simulink model "VSG_10k"  (R2022b)
settings: Solver=FixedStepAuto  StartTime=0.0  StopTime=4  FixedStep=1e-6  RelTol=1e-3
model workspace (MAT data in the model file):
  C = 0.0002
  D = 100
  GP = 1
  GQ = 3
  J = 5
  KQ = 0.06
  Kf = 120
  Kv = 577
  L = 0.002
  Pref = 10000
  Qref = 0
  Ts = 1e-06
  Ug = 563.38264084
  Vdc = 800
  fsw = 20000
  t0 = 0.5
  tco = 1.3
  tf = 1.2
  wn = 314.159265359
undefined symbols (not defined in the file): DiscIntNeverNeededParam
libraries: spsabctodq0Lib x4, spsPowerPositiveSequenceLib x4, slpidlib x4, spsFirstOrderFilterLib x3, spsMultimeterLib x3, spsThreePhaseSeriesRLCBranchLib x3, spsThreePhaseVIMeasurementLib x3, spsGroundLib x2, spsPLL3phLib x2, spsDCVoltageSourceLib x1, spsPWMGenerator2LevelLib x1, spsdq0toabcLib x1
settings Model: SimulationMode=accelerator  Creator=刘明炜  LastModifiedBy=user
settings DataIOCC: ReturnWorkspaceOutputs=off

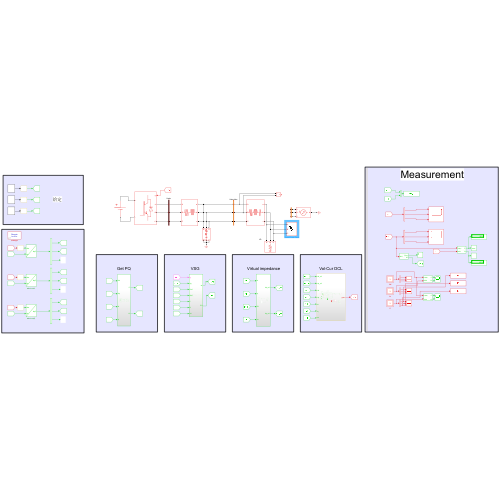
[thumbnail: Simulink's stored preview of the top-level diagram]
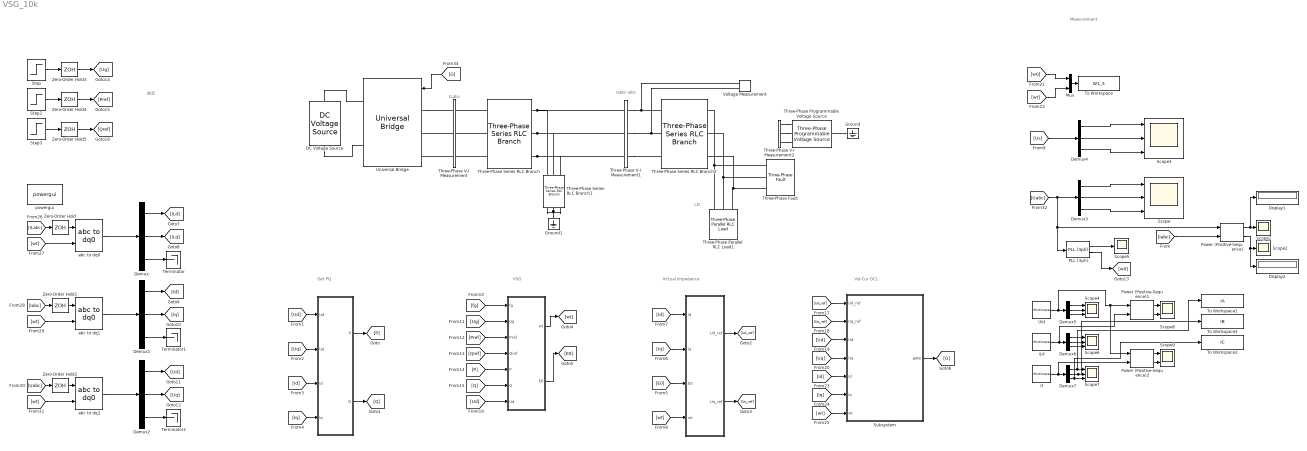
== system VSG_10k ==
  note: Measurement
  note: 给定
  note: ILabc
  note: VSG
  note: LD
  note: Get PQ
  note: Virtual impedance
  note: Vol-Cur DCL
  note: Uabc-Iabc
  " " : Subsystem
  "  " : Subsystem
  "   " : Subsystem
  DC Voltage Source : spsDCVoltageSourceLib/DC Voltage Source  Amplitude=1000  Measurements=None
  Demux{,1..7} (8 alike) : Demux  Outputs=3
  Display1 : Display
  Display2 : Display
  Ground : spsGroundLib/Ground  LConnTagsString=a
  Ground1 : spsGroundLib/Ground  LConnTagsString=a
  If : spsMultimeterLib/Multimeter  L=12  sel=[10 11 12]  yselected={}  Gain=[1 1 1]  OutputType=Complex  PlotAtSimulationStop=off  PhasorSimulation=off
  Mux : Mux  Inputs=2
  PLL (3ph) : spsPLL3phLib/PLL (3ph)  Fmin=45  Par_Init=[0, 50]  ParK=[180, 3200, 1]  TcD=1e-4  MaxRateChangeFreq=12  FilterCutOffFreq=25  Ts=1/fsw  AGC=on
  Power (Positive-Sequence) : spsPowerPositiveSequenceLib/Power (Positive-Sequence)  Freq=50  Vinit=[0, 0]  Iinit=[0, 0]  Ts=1/fsw
      settings: LibrarySourceBlock=|
      | sps_lib/Sensors and Measurements/Power
      | (Positive-Sequence)
  Power (Positive-Sequence)1 : spsPowerPositiveSequenceLib/Power (Positive-Sequence)  Freq=50  Vinit=[0, 0]  Iinit=[0, 0]  Ts=1/fsw
      settings: LibrarySourceBlock=|
      | sps_lib/Sensors and Measurements/Power
      | (Positive-Sequence)
  Power (Positive-Sequence)2 : spsPowerPositiveSequenceLib/Power (Positive-Sequence)  Freq=50  Vinit=[0, 0]  Iinit=[0, 0]  Ts=1/fsw
      settings: LibrarySourceBlock=|
      | sps_lib/Sensors and Measurements/Power
      | (Positive-Sequence)
  Scope{,3..4,6..7} (5 alike) : Scope  NumInputPorts=3
  Scope1 : Scope
  Scope2 : Scope
  Scope5 : Scope
  Scope8 : Scope  NumInputPorts=2
  Scope9 : Scope  NumInputPorts=2
  Step : Step  Time=0.5  Before=1  After=Ug  SampleTime=0
  Step1 : Step  Time=t0  After=Pref  SampleTime=0
  Step3 : Step  Time=t0  After=Qref  SampleTime=0
  Subsystem : Subsystem
  Terminator : Terminator
  Terminator1 : Terminator
  Terminator2 : Terminator
  Three-Phase Parallel RLC Load1 : spsThreePhaseParallelRLCLoadLib/Three-Phase Parallel RLC Load  LConnTagsString=A|B|C  Configuration=Y (grounded)  NominalVoltage=690  Vabc=[1e3 1e3 1e3]  Vabcp=[1e3 1e3 1e3]  NominalFrequency=50  UnbalancedPower=off  ActivePower=10e3  InductivePower=0  CapacitivePower=0  Pabc=[10e3 9e3 11e3]  QLabc=[100 90 110]  QCabc=[100 90 110]  Pabcp=[10e3 9e3 11e3]  QLabcp=[100 90 110]  QCabcp=[100 90 110]  Measurements=Branch voltages and currents  LoadType=constant Z
  Three-Phase Programmable Voltage Source : spsThreePhaseProgrammableVoltageSourceLib/Three-Phase Programmable Voltage Source  PositiveSequence="[690  0 50]"  VariationEntity=None  VariationType=Table of time-amplitude pairs  VariationTypeAlt=Step  VariationStep=0.5  VariationRate=10  VariationMagnitude=0.3  VariationFrequency=2  VariationTiming=[1 2]  VariationPhaseA=off  Amplitudes=[1 0.8 1.2 1.0]  TimeValues=[0 0.1 0.15 0.2]  HarmonicGeneration=off  HarmonicA=[3 0.2 -25 0]  HarmonicB=[2 0.15 35 2]  Timing="[0.05  3]"  BusType=PQ  Pref=-20000  Qref=0  Qmin=-inf  Qmax=inf
  Three-Phase Series RLC Branch : spsThreePhaseSeriesRLCBranchLib/Three-Phase Series RLC Branch  LConnTagsString=A|B|C  RConnTagsString=A|B|C  BranchType=RL  Resistance=0  Inductance=0.002  Capacitance=0  Measurements=None
  Three-Phase Series RLC Branch1 : spsThreePhaseSeriesRLCBranchLib/Three-Phase Series RLC Branch  LConnTagsString=A|B|C  RConnTagsString=A|B|C  BranchType=RLC  Resistance=1  Inductance=0  Capacitance=0.0002  Measurements=None
  Three-Phase Series RLC Branch2 : spsThreePhaseSeriesRLCBranchLib/Three-Phase Series RLC Branch  LConnTagsString=A|B|C  RConnTagsString=A|B|C  BranchType=RLC  Resistance=0  Inductance=7e-3  Capacitance=0  Measurements=None
  Three-Phase V-I Measurement : spsThreePhaseVIMeasurementLib/Three-Phase V-I Measurement  VoltageMeasurement=phase-to-phase  SetLabelV=on  LabelV=vnon  Vpu=off  VpuLL=off  CurrentMeasurement=yes  SetLabelI=on  LabelI=ILabc  Ipu=off  Pbase=100e6  Vbase=500e3  OutputType=Complex  PhasorSimulation=off  PSBequivalent=0
  Three-Phase V-I Measurement1 : spsThreePhaseVIMeasurementLib/Three-Phase V-I Measurement  VoltageMeasurement=phase-to-ground  SetLabelV=on  LabelV=Uabc  Vpu=off  VpuLL=off  CurrentMeasurement=yes  SetLabelI=on  LabelI=Iabc  Ipu=off  Pbase=100e6  Vbase=500e3  OutputType=Complex  PhasorSimulation=off  PSBequivalent=0
  Three-Phase V-I Measurement2 : spsThreePhaseVIMeasurementLib/Three-Phase V-I Measurement  VoltageMeasurement=phase-to-ground  SetLabelV=on  LabelV=Us  Vpu=off  VpuLL=off  CurrentMeasurement=yes  SetLabelI=on  LabelI=Is  Ipu=off  Pbase=100e6  Vbase=500e3  OutputType=Complex  PhasorSimulation=off  PSBequivalent=0
  Three-Phase Fault : spsThreePhaseFaultLib/Three-Phase Fault  InitialStates=0  FaultA=on  FaultB=off  FaultC=off  GroundFault=on  SwitchTimes="[tf  tco]"  External=off  SwitchStatus=NaN  FaultResistance=0.001  GroundResistance=0.01  SnubberResistance=1e6  SnubberCapacitance=inf  Measurements=Fault voltages and currents
  To Workspace : ToWorkspace  VariableName=W1_5  SaveFormat=Timeseries  SampleTime=-1
  To Workspace1 : ToWorkspace  VariableName=IA  SaveFormat=Timeseries  SampleTime=-1
  To Workspace2 : ToWorkspace  VariableName=IC  SaveFormat=Timeseries  SampleTime=-1
  To Workspace3 : ToWorkspace  VariableName=IB  SaveFormat=Timeseries  SampleTime=-1
  Uld : spsMultimeterLib/Multimeter  L=12  sel=[1 2 3]  yselected={}  Gain=[1 1 1]  OutputType=Complex  PlotAtSimulationStop=off  PhasorSimulation=off
  Universal Bridge : spsUniversalBridgeLib/Universal Bridge  Arms=3  SnubberResistance=1e5  SnubberCapacitance=inf  Device=IGBT / Diodes  Ron=0.001  Lon=0  ForwardVoltages="[  0  0  ]"  ForwardVoltage=0  GTOparameters=[ 10e-6 , 20e-6 ]  IGBTparameters=[ 1e-6 , 2e-6 ]  Measurements=None  Measurements_2=None  converterType=Rectifier
  Voltage Measurement : spsVoltageMeasurementLib/Voltage Measurement  PhasorSimulation=off  OutputType=Complex  PSBequivalent=0
  Zero-Order Hold{,1..5} (6 alike) : ZeroOrderHold  SampleTime=1/fsw
  abc to dq0 : spsabctodq0Lib/abc to dq0  Alignment=90 degrees behind phase A axis
  abc to dq1 : spsabctodq0Lib/abc to dq0  Alignment=90 degrees behind phase A axis
  abc to dq2 : spsabctodq0Lib/abc to dq0  Alignment=90 degrees behind phase A axis
  iLd : spsMultimeterLib/Multimeter  L=12  sel=[7 8 9]  yselected={}  Gain=[1 1 1]  OutputType=Complex  PlotAtSimulationStop=off  PhasorSimulation=off
  powergui : sps_lib/powergui  Priority=1  SimulationMode=Discrete  SampleTime=1e-6  frequency=60  Iterations=50  frequencyindice=0  Pbase=100e6  ErrMax=1e-4  UnitsV=kV  UnitsW=MW  buscounter=0  FunctionMessages=off  echomessages=off  EnableUseOfTLC=off  CurrentSourceSwitches=off  DisableSnubberDevices=off  DisableRonSwitches=off  DisableVfSwitches=off  DisplayEquations=off  AutomaticDiscreteSolvers=off  SolverType=Tustin/Backward Euler (TBE)  Interpol=off  ExternalGateDelay=off  methode=off  Ts=100  x0status=blocks  SPID=on  SwTol=0  HookPort=off  NonlinearTolerance=1e-4  nMaxIteration=100  ContinueOnMaxIteration=off  RestoreLinks=warning  ResistiveCurrentMeasurement=off  Frange=[0:2:500]  Ylog=off  Xlog=on  ShowGrid=off  save=off  variable=ZData  structure=0  ZoomFFT=off  StartTime=0.0  cycles=1  DisplayStyle=1  fundamental=60  FreqAxis=off  MaxFrequency=1000  frequencyindicesteady=1  RmsSteady=1  display=off
  wires:
  [Id] -> " "/3(Id)
  [Iq] -> " "/4(Iq)
  [Uq] -> " "/2(Uq)
  " "/1(P) -> [P]
  [Ud] -> " "/1(Ud)
  " "/2(Q) -> [Q]
  [E0] -> "   "/3(E0)
  [Iq] -> "   "/2(Iq)
  [Id] -> "   "/1(Id)
  [wt] -> "   "/4(wt)
  "   "/1(Ud_ref) -> [Ud_ref]
  "   "/2(Uq_ref) -> [Uq_ref]
  [Qref] -> "  "/4(Qref)
  [Ud] -> "  "/7(Ud)
  [fg] -> "  "/1(fg)
  "  "/2(E0) -> [E0]
  [Q] -> "  "/6(Q)
  [P] -> "  "/5(P)
  [Ug] -> "  "/2(Ug)
  [Pref] -> "  "/3(Pref)
  "  "/1(wt) -> [wt]
  [Ud] -> Subsystem/3(Ud)
  Subsystem/1(gate) -> [G]
  [wt] -> Subsystem/7(wt)
  [Ud_ref] -> Subsystem/1(Ud_ref)
  [Uq_ref] -> Subsystem/2(Uq_ref)
  [Iq] -> Subsystem/6(Iq)
  [Uq] -> Subsystem/4(Uq)
  [Id] -> Subsystem/5(Id)
  abc to dq0/1 -> Demux/1
  Demux/1 -> [ILd]
  Demux/2 -> [ILq]
  Demux/3 -> Terminator/1
  Demux1/2 -> [Iq]
  Demux1/1 -> [Id]
  abc to dq1/1 -> Demux1/1
  Demux1/3 -> Terminator1/1
  Demux2/2 -> [Uq]
  Demux2/1 -> [Ud]
  abc to dq2/1 -> Demux2/1
  Demux2/3 -> Terminator2/1
  Zero-Order Hold/1 -> abc to dq0/1
  [ILabc] -> Zero-Order Hold/1
  [Iabc] -> Zero-Order Hold1/1
  Zero-Order Hold1/1 -> abc to dq1/1
  [Uabc] -> Zero-Order Hold2/1
  Zero-Order Hold2/1 -> abc to dq2/1
  [wt] -> abc to dq0/2
  [wt] -> abc to dq1/2
  [wt] -> abc to dq2/2
  Step/1 -> Zero-Order Hold3/1
  Zero-Order Hold3/1 -> [Ug]
  Zero-Order Hold4/1 -> [Pref]
  Step1/1 -> Zero-Order Hold4/1
  [Uabc] -> PLL (3ph)/1, Power (Positive-Sequence)/1, Demux3/1
  Demux3/1 -> Scope/1
  Demux3/2 -> Scope/2
  Demux3/3 -> Scope/3
  [G] -> Universal Bridge/1
  [Iabc] -> Power (Positive-Sequence)/2
  Power (Positive-Sequence)/1 -> Display1/1, Scope1/1
  Power (Positive-Sequence)/2 -> Display2/1, Scope2/1
  Step3/1 -> Zero-Order Hold5/1
  Zero-Order Hold5/1 -> [Qref]
  Demux4/2 -> Scope3/2
  Demux4/3 -> Scope3/3
  [Us] -> Demux4/1
  Demux4/1 -> Scope3/1
  PLL (3ph)/1 -> Scope5/1
  PLL (3ph)/2 -> [w0]
  [w0] -> Mux/1
  [wt] -> Mux/2
  Mux/1 -> To Workspace/1
  Uld/1 -> Power (Positive-Sequence)2/1, Power (Positive-Sequence)1/1, Demux5/1
  iLd/1 -> Power (Positive-Sequence)1/2, Demux6/1
  If/1 -> Power (Positive-Sequence)2/2, Demux7/1
  Demux5/1 -> Scope4/1
  Demux5/2 -> Scope4/2
  Demux5/3 -> Scope4/3
  Demux6/1 -> Scope6/1
  Demux6/2 -> Scope6/2
  Demux6/3 -> Scope6/3
  Demux7/1 -> To Workspace1/1, Scope7/1
  Demux7/2 -> To Workspace3/1, Scope7/2
  Demux7/3 -> To Workspace2/1, Scope7/3
  Power (Positive-Sequence)1/1 -> Scope8/1
  Power (Positive-Sequence)1/2 -> Scope8/2
  Power (Positive-Sequence)2/1 -> Scope9/1
  Power (Positive-Sequence)2/2 -> Scope9/2
  connections:
  Three-Phase Series RLC Branch/RConn1 -- Three-Phase V-I Measurement1/LConn1 -- Three-Phase Series RLC Branch1/LConn1
  Ground1/LConn1 -- Three-Phase Series RLC Branch1/RConn2 -- Three-Phase Series RLC Branch1/RConn3 -- Three-Phase Series RLC Branch1/RConn1
  Three-Phase Series RLC Branch/RConn3 -- Three-Phase V-I Measurement1/LConn3 -- Three-Phase Series RLC Branch1/LConn3
  Three-Phase Series RLC Branch/RConn2 -- Three-Phase Series RLC Branch1/LConn2 -- Three-Phase V-I Measurement1/LConn2
  Three-Phase Series RLC Branch/LConn1 -- Three-Phase V-I Measurement/RConn1
  Three-Phase V-I Measurement1/RConn3 -- Three-Phase Series RLC Branch2/LConn3
  Three-Phase V-I Measurement/LConn2 -- Universal Bridge/LConn2
  DC Voltage Source/LConn1 -- Universal Bridge/RConn2
  Universal Bridge/LConn1 -- Three-Phase V-I Measurement/LConn1
  Three-Phase V-I Measurement1/RConn2 -- Voltage Measurement/LConn2 -- Three-Phase Series RLC Branch2/LConn2
  DC Voltage Source/RConn1 -- Universal Bridge/RConn1
  Three-Phase V-I Measurement1/RConn1 -- Voltage Measurement/LConn1 -- Three-Phase Series RLC Branch2/LConn1
  Three-Phase Series RLC Branch/LConn2 -- Three-Phase V-I Measurement/RConn2
  Three-Phase Series RLC Branch/LConn3 -- Three-Phase V-I Measurement/RConn3
  Three-Phase V-I Measurement/LConn3 -- Universal Bridge/LConn3
  Ground/LConn1 -- Three-Phase Programmable Voltage Source/LConn1
  Three-Phase V-I Measurement2/RConn1 -- Three-Phase Programmable Voltage Source/RConn1
  Three-Phase V-I Measurement2/RConn2 -- Three-Phase Programmable Voltage Source/RConn2
  Three-Phase V-I Measurement2/RConn3 -- Three-Phase Programmable Voltage Source/RConn3
  Three-Phase Parallel RLC Load1/LConn1 -- Three-Phase Fault/LConn1 -- Three-Phase Series RLC Branch2/RConn1
  Three-Phase Parallel RLC Load1/LConn3 -- Three-Phase Series RLC Branch2/RConn3 -- Three-Phase Fault/LConn3
  Three-Phase Fault/LConn2 -- Three-Phase Series RLC Branch2/RConn2 -- Three-Phase Parallel RLC Load1/LConn2

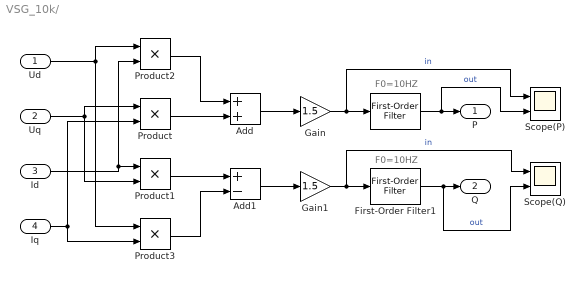
== system VSG_10k/  ==
  note: F0=10HZ
  note: F0=10HZ
  Ud : Inport
  Uq : Inport  Port=2
  Id : Inport  Port=3
  Iq : Inport  Port=4
  " " : spsFirstOrderFilterLib/First-Order Filter  FilterType=Lowpass  Tc=10e-3  Ts=1/fsw  Initialize=on  Vac_Init=[0, 0, 10]  Vdc_Init=0  PlotResponse=off  FreqRange="[0,  200,  1]"
  Add : Sum
  Add1 : Sum  Inputs=+-
  First-Order Filter1 : spsFirstOrderFilterLib/First-Order Filter  FilterType=Lowpass  Tc=10e-3  Ts=1/fsw  Initialize=on  Vac_Init=[0, 0, 10]  Vdc_Init=0  PlotResponse=off  FreqRange="[0,  200,  1]"
  Gain : Gain  Gain=1.5
  Gain1 : Gain  Gain=1.5
  Product{,1..3} (4 alike) : Product
  Scope(P) : Scope  NumInputPorts=2
  Scope(Q) : Scope  NumInputPorts=2
  P : Outport
  Q : Outport  Port=2
  wires:
  Gain1/1 -> First-Order Filter1/1, Scope(Q)/1  "in"
  Product2/1 -> Add/1
  " "/1 -> Scope(P)/2, P/1  "out"
  Add1/1 -> Gain1/1
  Gain/1 -> " "/1, Scope(P)/1  "in"
  First-Order Filter1/1 -> Scope(Q)/2, Q/1  "out"
  Product/1 -> Add/2
  Product3/1 -> Add1/2
  Product1/1 -> Add1/1
  Ud/1 -> Product3/1, Product2/1
  Add/1 -> Gain/1
  Id/1 -> Product1/1, Product2/2
  Iq/1 -> Product3/2, Product/2
  Uq/1 -> Product1/2, Product/1

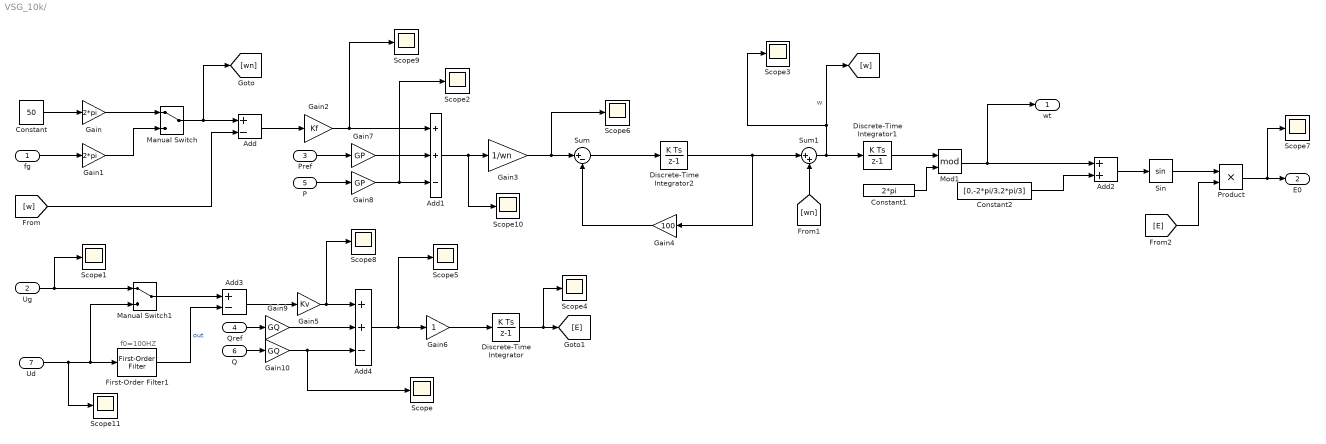
== system VSG_10k/   ==
  note: f0=100HZ
  note: w
  fg : Inport
  Ug : Inport  Port=2
  Pref : Inport  Port=3
  Qref : Inport  Port=4
  P : Inport  Port=5
  Q : Inport  Port=6
  Ud : Inport  Port=7
  Add : Sum  Inputs=+-
  Add1 : Sum  Inputs=++-
  Add2 : Sum
  Add3 : Sum  Inputs=+-
  Add4 : Sum  Inputs=++-
  Constant : Constant  Value=50
  Constant1 : Constant  Value=2*pi
  Constant2 : Constant  Value=[0,-2*pi/3,2*pi/3]
  Discrete-Time Integrator : DiscreteIntegrator  gainval=KQ  SampleTime=1/fsw  ICPrevOutput=DiscIntNeverNeededParam  ICPrevScaledInput=DiscIntNeverNeededParam
  Discrete-Time Integrator1 : DiscreteIntegrator  SampleTime=1/fsw  ICPrevOutput=DiscIntNeverNeededParam  ICPrevScaledInput=DiscIntNeverNeededParam
  Discrete-Time Integrator2 : DiscreteIntegrator  gainval=1/J  SampleTime=1/fsw  ICPrevOutput=DiscIntNeverNeededParam  ICPrevScaledInput=DiscIntNeverNeededParam
  First-Order Filter1 : spsFirstOrderFilterLib/First-Order Filter  FilterType=Lowpass  Tc=10e-3  Ts=1/fsw  Initialize=on  Vac_Init=[0, 0, 10]  Vdc_Init=0  PlotResponse=off  FreqRange="[0,  200,  1]"
  Gain : Gain  Gain=2*pi
  Gain1 : Gain  Gain=2*pi
  Gain10 : Gain  Gain=GQ
  Gain2 : Gain  Gain=Kf
  Gain3 : Gain  Gain=1/wn
  Gain4 : Gain  Gain=100
  Gain5 : Gain  Gain=Kv
  Gain6 : Gain
  Gain7 : Gain  Gain=GP
  Gain8 : Gain  Gain=GP
  Gain9 : Gain  Gain=GQ
  Manual Switch : ManualSwitch
  Manual Switch1 : ManualSwitch
  Mod1 : Math  Operator=mod
  Product : Product
  Scope{,1..11} (12 alike) : Scope
  Sin : Trigonometry
  Sum : Sum  Inputs=|+-
  Sum1 : Sum  Inputs=|++
  wt : Outport
  E0 : Outport  Port=2
  wires:
  Ug/1 -> Scope1/1, Manual Switch1/1
  Gain3/1 -> Scope6/1, Sum/1
  Gain2/1 -> Scope9/1, Add1/1
  Product/1 -> Scope7/1, E0/1
  Add/1 -> Gain2/1
  Manual Switch1/1 -> Add3/1
  [E] -> Product/2
  Add4/1 -> Scope5/1, Gain6/1
  Mod1/1 -> wt/1, Add2/1
  Sum1/1 -> Discrete-Time Integrator1/1, Scope3/1, [w]
  fg/1 -> Gain1/1
  Constant2/1 -> Add2/2
  First-Order Filter1/1 -> Add3/2  "out"
  Constant/1 -> Gain/1
  Sin/1 -> Product/1
  Add2/1 -> Sin/1
  Gain4/1 -> Sum/2
  P/1 -> Gain8/1
  Gain/1 -> Manual Switch/1
  Gain1/1 -> Manual Switch/2
  Discrete-Time Integrator2/1 -> Gain4/1, Sum1/1
  Constant1/1 -> Mod1/2
  Gain5/1 -> Scope8/1, Add4/1
  Q/1 -> Gain10/1
  Manual Switch/1 -> [wn], Add/1
  Pref/1 -> Gain7/1
  Add1/1 -> Scope10/1, Gain3/1
  Add3/1 -> Gain5/1
  Gain6/1 -> Discrete-Time Integrator/1
  Qref/1 -> Gain9/1
  [wn] -> Sum1/2
  Sum/1 -> Discrete-Time Integrator2/1
  Discrete-Time Integrator/1 -> Scope4/1, [E]
  Discrete-Time Integrator1/1 -> Mod1/1
  [w] -> Add/2
  Gain7/1 -> Add1/2
  Gain8/1 -> Scope2/1, Add1/3
  Gain9/1 -> Add4/2
  Gain10/1 -> Scope/1, Add4/3
  Ud/1 -> Scope11/1, First-Order Filter1/1, Manual Switch1/2

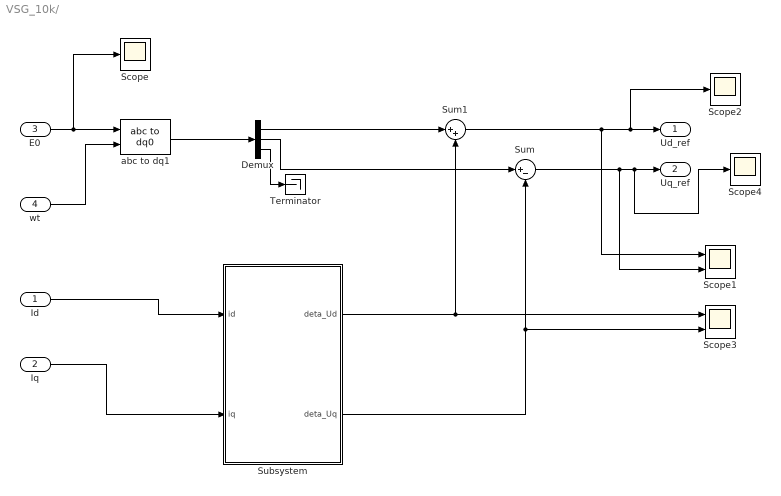
== system VSG_10k/    ==
  Id : Inport
  Iq : Inport  Port=2
  E0 : Inport  Description=Cont  Port=3
  wt : Inport  Port=4
  Demux : Demux  Outputs=3
  Scope : Scope
  Scope1 : Scope  NumInputPorts=2
  Scope2 : Scope
  Scope3 : Scope  NumInputPorts=2
  Scope4 : Scope
  Subsystem : Subsystem
  Sum : Sum  Inputs=|+-
  Sum1 : Sum  Inputs=|++
  Terminator : Terminator
  abc to dq1 : spsabctodq0Lib/abc to dq0  Alignment=90 degrees behind phase A axis
  Ud_ref : Outport
  Uq_ref : Outport  Port=2
  wires:
  Demux/1 -> Sum1/1
  E0/1 -> Scope/1, abc to dq1/1
  Id/1 -> Subsystem/1(id)
  abc to dq1/1 -> Demux/1
  Subsystem/2(deta_Uq) -> Scope3/2, Sum/2
  Sum1/1 -> Scope2/1, Ud_ref/1, Scope1/1
  wt/1 -> abc to dq1/2
  Demux/2 -> Sum/1
  Subsystem/1(deta_Ud) -> Sum1/2, Scope3/1
  Iq/1 -> Subsystem/2(iq)
  Sum/1 -> Scope4/1, Uq_ref/1, Scope1/2
  Demux/3 -> Terminator/1

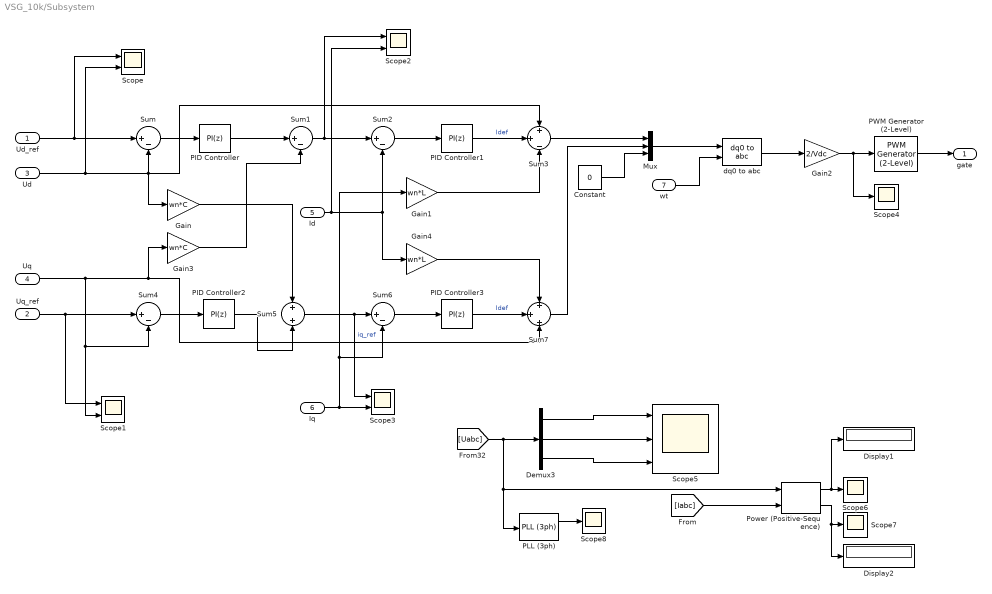
== system VSG_10k/Subsystem ==
  Ud_ref : Inport
  Uq_ref : Inport  Port=2
  Ud : Inport  Port=3
  Uq : Inport  Port=4
  Id : Inport  Port=5
  Iq : Inport  Port=6
  wt : Inport  Port=7
  Constant : Constant  Value=0
  Demux3 : Demux  Outputs=3
  Display1 : Display
  Display2 : Display
  Gain : Gain  Gain=wn*C
  Gain1 : Gain  Gain=wn*L
  Gain2 : Gain  Gain=2/Vdc
  Gain3 : Gain  Gain=wn*C
  Gain4 : Gain  Gain=wn*L
  Mux : Mux  Inputs=3
  PID Controller : slpidlib/PID Controller  Controller=PI  Form=Parallel  TimeDomain=Discrete-time  UseExternalTs=off  SampleTime=-1  IntegratorMethod=Forward Euler  FilterMethod=Forward Euler  ControllerParametersSource=internal  P=10  I=50  UseKiTs=off  D=0  N=100  UseFilter=on  TunerSelectOption=Transfer Function Based (PID Tuner App)  InitialConditionSource=internal  InitialConditionForIntegrator=0  InitialConditionForFilter=0  DifferentiatorICPrevScaledInput=0  ExternalReset=none  TrackingMode=off  Kt=1  LimitOutput=off  SatLimitsSource=internal  UpperSaturationLimit=inf  LowerSaturationLimit=-inf  LinearizeAsGain=on  AntiWindupMode=none  Kb=1  LimitIntegrator=off  UpperIntegratorSaturationLimit=inf  LowerIntegratorSaturationLimit=-inf  POutMin=[]  POutMax=[]  IOutMin=[]  IOutMax=[]  DOutMin=[]  DOutMax=[]  NOutMin=[]  NOutMax=[]  SumOutMin=[]  SumOutMax=[]  SaturationOutMin=[]  SaturationOutMax=[]  PParamMin=[]  PParamMax=[]  IParamMin=[]  IParamMax=[]  DParamMin=[]  DParamMax=[]  NParamMin=[]  NParamMax=[]  KbParamMin=[]  KbParamMax=[]  KtParamMin=[]  KtParamMax=[]  KbOutMin=[]  KbOutMax=[]  KtOutMin=[]  KtOutMax=[]  IntegratorOutMin=[]  IntegratorOutMax=[]  FilterOutMin=[]  FilterOutMax=[]  SumI1OutMin=[]  SumI1OutMax=[]  SumI2OutMin=[]  SumI2OutMax=[]  SumI3OutMin=[]  SumI3OutMax=[]  SumI4OutMin=[]  SumI4OutMax=[]  SumDOutMin=[]  SumDOutMax=[]  DifferentiatorOutMin=[]  DifferentiatorOutMax=[]  FilterDiffOutCoefMin=[]  FilterDiffOutCoefMax=[]  ReciprocalOutMin=[]  ReciprocalOutMax=[]  SumDenOutMin=[]  SumDenOutMax=[]  SumNumOutMin=[]  SumNumOutMax=[]  DivideOutMin=[]  DivideOutMax=[]  UdiffTsProdOutMin=[]  UdiffTsProdOutMax=[]  NTsProdOutMin=[]  NTsProdOutMax=[]  UintegralTsProdOutMin=[]  UintegralTsProdOutMax=[]  UngainTsProdOutMin=[]  UngainTsProdOutMax=[]  ClampingZeroOutDataTypeStr=Inherit: Inherit via back propagation  ClampingZeroOutMin=[]  ClampingZeroOutMax=[]  FilterDenConstantOutDataTypeStr=Inherit: Inherit via back propagation  FilterDenConstantOutMin=[]  FilterDenConstantOutMax=[]  PCopyOutDataTypeStr=Inherit: Inherit via back propagation  PCopyOutMin=[]  PCopyOutMax=[]  NCopyOutDataTypeStr=Inherit: Inherit via back propagation  NCopyOutMin=[]  NCopyOutMax=[]  IntegratorContinuousStateAttributes=''  IntegratorStateMustResolveToSignalObject=off  IntegratorRTWStateStorageClass=Auto  FilterContinuousStateAttributes=''  FilterStateMustResolveToSignalObject=off  FilterRTWStateStorageClass=Auto  ParallelPVariant=InternalParameters  IdealPVariant=Disabled  IVariant=InternalParameters  DVariant=Disabled  IntegratorVariant=Discrete  SatVariant=Disabled  AWVariant=Passthrough  PCopyVariant=Disabled  TRVariant=Disabled  FdbkBlocksVariant=Forward  IdealPFdbkVariant=Disabled  SatFdbkVariant=Disabled  DerivativeFilterVariant=Disabled  NVariant=Disabled  NCopyVariant=Disabled_SignalSpec  FilterICVariant=Disabled  IntegratorICVariant=InternalICs  ExternalResetVariant=Disabled  TRSumVariant=Passthrough  SumFdbkVariant=Disabled  SumVariant=Sum_PI  TsampFilterVariant=InternalTs  TsampNgainVariant=Passthrough  TsampIntegralVariant=Passthrough  ExternalSaturationOutDataTypeStr=Inherit: Same as second input
  PID Controller1 : slpidlib/PID Controller  Controller=PI  Form=Parallel  TimeDomain=Discrete-time  UseExternalTs=off  SampleTime=-1  IntegratorMethod=Forward Euler  FilterMethod=Forward Euler  ControllerParametersSource=internal  P=20  I=50  UseKiTs=off  D=0  N=100  UseFilter=on  TunerSelectOption=Transfer Function Based (PID Tuner App)  InitialConditionSource=internal  InitialConditionForIntegrator=0  InitialConditionForFilter=0  DifferentiatorICPrevScaledInput=0  ExternalReset=none  TrackingMode=off  Kt=1  LimitOutput=off  SatLimitsSource=internal  UpperSaturationLimit=inf  LowerSaturationLimit=-inf  LinearizeAsGain=on  AntiWindupMode=none  Kb=1  LimitIntegrator=off  UpperIntegratorSaturationLimit=inf  LowerIntegratorSaturationLimit=-inf  POutMin=[]  POutMax=[]  IOutMin=[]  IOutMax=[]  DOutMin=[]  DOutMax=[]  NOutMin=[]  NOutMax=[]  SumOutMin=[]  SumOutMax=[]  SaturationOutMin=[]  SaturationOutMax=[]  PParamMin=[]  PParamMax=[]  IParamMin=[]  IParamMax=[]  DParamMin=[]  DParamMax=[]  NParamMin=[]  NParamMax=[]  KbParamMin=[]  KbParamMax=[]  KtParamMin=[]  KtParamMax=[]  KbOutMin=[]  KbOutMax=[]  KtOutMin=[]  KtOutMax=[]  IntegratorOutMin=[]  IntegratorOutMax=[]  FilterOutMin=[]  FilterOutMax=[]  SumI1OutMin=[]  SumI1OutMax=[]  SumI2OutMin=[]  SumI2OutMax=[]  SumI3OutMin=[]  SumI3OutMax=[]  SumI4OutMin=[]  SumI4OutMax=[]  SumDOutMin=[]  SumDOutMax=[]  DifferentiatorOutMin=[]  DifferentiatorOutMax=[]  FilterDiffOutCoefMin=[]  FilterDiffOutCoefMax=[]  ReciprocalOutMin=[]  ReciprocalOutMax=[]  SumDenOutMin=[]  SumDenOutMax=[]  SumNumOutMin=[]  SumNumOutMax=[]  DivideOutMin=[]  DivideOutMax=[]  UdiffTsProdOutMin=[]  UdiffTsProdOutMax=[]  NTsProdOutMin=[]  NTsProdOutMax=[]  UintegralTsProdOutMin=[]  UintegralTsProdOutMax=[]  UngainTsProdOutMin=[]  UngainTsProdOutMax=[]  ClampingZeroOutDataTypeStr=Inherit: Inherit via back propagation  ClampingZeroOutMin=[]  ClampingZeroOutMax=[]  FilterDenConstantOutDataTypeStr=Inherit: Inherit via back propagation  FilterDenConstantOutMin=[]  FilterDenConstantOutMax=[]  PCopyOutDataTypeStr=Inherit: Inherit via back propagation  PCopyOutMin=[]  PCopyOutMax=[]  NCopyOutDataTypeStr=Inherit: Inherit via back propagation  NCopyOutMin=[]  NCopyOutMax=[]  IntegratorContinuousStateAttributes=''  IntegratorStateMustResolveToSignalObject=off  IntegratorRTWStateStorageClass=Auto  FilterContinuousStateAttributes=''  FilterStateMustResolveToSignalObject=off  FilterRTWStateStorageClass=Auto  ParallelPVariant=InternalParameters  IdealPVariant=Disabled  IVariant=InternalParameters  DVariant=Disabled  IntegratorVariant=Discrete  SatVariant=Disabled  AWVariant=Passthrough  PCopyVariant=Disabled  TRVariant=Disabled  FdbkBlocksVariant=Forward  IdealPFdbkVariant=Disabled  SatFdbkVariant=Disabled  DerivativeFilterVariant=Disabled  NVariant=Disabled  NCopyVariant=Disabled_SignalSpec  FilterICVariant=Disabled  IntegratorICVariant=InternalICs  ExternalResetVariant=Disabled  TRSumVariant=Passthrough  SumFdbkVariant=Disabled  SumVariant=Sum_PI  TsampFilterVariant=InternalTs  TsampNgainVariant=Passthrough  TsampIntegralVariant=Passthrough  ExternalSaturationOutDataTypeStr=Inherit: Same as second input
  PID Controller2 : slpidlib/PID Controller  Controller=PI  Form=Parallel  TimeDomain=Discrete-time  UseExternalTs=off  SampleTime=-1  IntegratorMethod=Forward Euler  FilterMethod=Forward Euler  ControllerParametersSource=internal  P=10  I=50  UseKiTs=off  D=0  N=100  UseFilter=on  TunerSelectOption=Transfer Function Based (PID Tuner App)  InitialConditionSource=internal  InitialConditionForIntegrator=0  InitialConditionForFilter=0  DifferentiatorICPrevScaledInput=0  ExternalReset=none  TrackingMode=off  Kt=1  LimitOutput=off  SatLimitsSource=internal  UpperSaturationLimit=inf  LowerSaturationLimit=-inf  LinearizeAsGain=on  AntiWindupMode=none  Kb=1  LimitIntegrator=off  UpperIntegratorSaturationLimit=inf  LowerIntegratorSaturationLimit=-inf  POutMin=[]  POutMax=[]  IOutMin=[]  IOutMax=[]  DOutMin=[]  DOutMax=[]  NOutMin=[]  NOutMax=[]  SumOutMin=[]  SumOutMax=[]  SaturationOutMin=[]  SaturationOutMax=[]  PParamMin=[]  PParamMax=[]  IParamMin=[]  IParamMax=[]  DParamMin=[]  DParamMax=[]  NParamMin=[]  NParamMax=[]  KbParamMin=[]  KbParamMax=[]  KtParamMin=[]  KtParamMax=[]  KbOutMin=[]  KbOutMax=[]  KtOutMin=[]  KtOutMax=[]  IntegratorOutMin=[]  IntegratorOutMax=[]  FilterOutMin=[]  FilterOutMax=[]  SumI1OutMin=[]  SumI1OutMax=[]  SumI2OutMin=[]  SumI2OutMax=[]  SumI3OutMin=[]  SumI3OutMax=[]  SumI4OutMin=[]  SumI4OutMax=[]  SumDOutMin=[]  SumDOutMax=[]  DifferentiatorOutMin=[]  DifferentiatorOutMax=[]  FilterDiffOutCoefMin=[]  FilterDiffOutCoefMax=[]  ReciprocalOutMin=[]  ReciprocalOutMax=[]  SumDenOutMin=[]  SumDenOutMax=[]  SumNumOutMin=[]  SumNumOutMax=[]  DivideOutMin=[]  DivideOutMax=[]  UdiffTsProdOutMin=[]  UdiffTsProdOutMax=[]  NTsProdOutMin=[]  NTsProdOutMax=[]  UintegralTsProdOutMin=[]  UintegralTsProdOutMax=[]  UngainTsProdOutMin=[]  UngainTsProdOutMax=[]  ClampingZeroOutDataTypeStr=Inherit: Inherit via back propagation  ClampingZeroOutMin=[]  ClampingZeroOutMax=[]  FilterDenConstantOutDataTypeStr=Inherit: Inherit via back propagation  FilterDenConstantOutMin=[]  FilterDenConstantOutMax=[]  PCopyOutDataTypeStr=Inherit: Inherit via back propagation  PCopyOutMin=[]  PCopyOutMax=[]  NCopyOutDataTypeStr=Inherit: Inherit via back propagation  NCopyOutMin=[]  NCopyOutMax=[]  IntegratorContinuousStateAttributes=''  IntegratorStateMustResolveToSignalObject=off  IntegratorRTWStateStorageClass=Auto  FilterContinuousStateAttributes=''  FilterStateMustResolveToSignalObject=off  FilterRTWStateStorageClass=Auto  ParallelPVariant=InternalParameters  IdealPVariant=Disabled  IVariant=InternalParameters  DVariant=Disabled  IntegratorVariant=Discrete  SatVariant=Disabled  AWVariant=Passthrough  PCopyVariant=Disabled  TRVariant=Disabled  FdbkBlocksVariant=Forward  IdealPFdbkVariant=Disabled  SatFdbkVariant=Disabled  DerivativeFilterVariant=Disabled  NVariant=Disabled  NCopyVariant=Disabled_SignalSpec  FilterICVariant=Disabled  IntegratorICVariant=InternalICs  ExternalResetVariant=Disabled  TRSumVariant=Passthrough  SumFdbkVariant=Disabled  SumVariant=Sum_PI  TsampFilterVariant=InternalTs  TsampNgainVariant=Passthrough  TsampIntegralVariant=Passthrough  ExternalSaturationOutDataTypeStr=Inherit: Same as second input
  PID Controller3 : slpidlib/PID Controller  Controller=PI  Form=Parallel  TimeDomain=Discrete-time  UseExternalTs=off  SampleTime=-1  IntegratorMethod=Forward Euler  FilterMethod=Forward Euler  ControllerParametersSource=internal  P=20  I=50  UseKiTs=off  D=0  N=100  UseFilter=on  TunerSelectOption=Transfer Function Based (PID Tuner App)  InitialConditionSource=internal  InitialConditionForIntegrator=0  InitialConditionForFilter=0  DifferentiatorICPrevScaledInput=0  ExternalReset=none  TrackingMode=off  Kt=1  LimitOutput=off  SatLimitsSource=internal  UpperSaturationLimit=inf  LowerSaturationLimit=-inf  LinearizeAsGain=on  AntiWindupMode=none  Kb=1  LimitIntegrator=off  UpperIntegratorSaturationLimit=inf  LowerIntegratorSaturationLimit=-inf  POutMin=[]  POutMax=[]  IOutMin=[]  IOutMax=[]  DOutMin=[]  DOutMax=[]  NOutMin=[]  NOutMax=[]  SumOutMin=[]  SumOutMax=[]  SaturationOutMin=[]  SaturationOutMax=[]  PParamMin=[]  PParamMax=[]  IParamMin=[]  IParamMax=[]  DParamMin=[]  DParamMax=[]  NParamMin=[]  NParamMax=[]  KbParamMin=[]  KbParamMax=[]  KtParamMin=[]  KtParamMax=[]  KbOutMin=[]  KbOutMax=[]  KtOutMin=[]  KtOutMax=[]  IntegratorOutMin=[]  IntegratorOutMax=[]  FilterOutMin=[]  FilterOutMax=[]  SumI1OutMin=[]  SumI1OutMax=[]  SumI2OutMin=[]  SumI2OutMax=[]  SumI3OutMin=[]  SumI3OutMax=[]  SumI4OutMin=[]  SumI4OutMax=[]  SumDOutMin=[]  SumDOutMax=[]  DifferentiatorOutMin=[]  DifferentiatorOutMax=[]  FilterDiffOutCoefMin=[]  FilterDiffOutCoefMax=[]  ReciprocalOutMin=[]  ReciprocalOutMax=[]  SumDenOutMin=[]  SumDenOutMax=[]  SumNumOutMin=[]  SumNumOutMax=[]  DivideOutMin=[]  DivideOutMax=[]  UdiffTsProdOutMin=[]  UdiffTsProdOutMax=[]  NTsProdOutMin=[]  NTsProdOutMax=[]  UintegralTsProdOutMin=[]  UintegralTsProdOutMax=[]  UngainTsProdOutMin=[]  UngainTsProdOutMax=[]  ClampingZeroOutDataTypeStr=Inherit: Inherit via back propagation  ClampingZeroOutMin=[]  ClampingZeroOutMax=[]  FilterDenConstantOutDataTypeStr=Inherit: Inherit via back propagation  FilterDenConstantOutMin=[]  FilterDenConstantOutMax=[]  PCopyOutDataTypeStr=Inherit: Inherit via back propagation  PCopyOutMin=[]  PCopyOutMax=[]  NCopyOutDataTypeStr=Inherit: Inherit via back propagation  NCopyOutMin=[]  NCopyOutMax=[]  IntegratorContinuousStateAttributes=''  IntegratorStateMustResolveToSignalObject=off  IntegratorRTWStateStorageClass=Auto  FilterContinuousStateAttributes=''  FilterStateMustResolveToSignalObject=off  FilterRTWStateStorageClass=Auto  ParallelPVariant=InternalParameters  IdealPVariant=Disabled  IVariant=InternalParameters  DVariant=Disabled  IntegratorVariant=Discrete  SatVariant=Disabled  AWVariant=Passthrough  PCopyVariant=Disabled  TRVariant=Disabled  FdbkBlocksVariant=Forward  IdealPFdbkVariant=Disabled  SatFdbkVariant=Disabled  DerivativeFilterVariant=Disabled  NVariant=Disabled  NCopyVariant=Disabled_SignalSpec  FilterICVariant=Disabled  IntegratorICVariant=InternalICs  ExternalResetVariant=Disabled  TRSumVariant=Passthrough  SumFdbkVariant=Disabled  SumVariant=Sum_PI  TsampFilterVariant=InternalTs  TsampNgainVariant=Passthrough  TsampIntegralVariant=Passthrough  ExternalSaturationOutDataTypeStr=Inherit: Same as second input
  PLL (3ph) : spsPLL3phLib/PLL (3ph)  Fmin=45  Par_Init=[0, 50]  ParK=[180, 3200, 1]  TcD=1e-4  MaxRateChangeFreq=12  FilterCutOffFreq=25  Ts=1/fsw  AGC=on
  PWM Generator (2-Level) : spsPWMGenerator2LevelLib/PWM Generator (2-Level)  ModulatorType=Three-phase bridge (6 pulses)  ModulatorMode=Unsynchronized  Fc=fsw  Pc=90  nF=27  MinMax="[ -1  1 ]"  SamplingTechnique=Natural  ModulatingSignals=off  m=0.8  Freq=60  Phase=0  Ts=Ts  ShowCarrierOutport=off
  Power (Positive-Sequence) : spsPowerPositiveSequenceLib/Power (Positive-Sequence)  Freq=50  Vinit=[0, 0]  Iinit=[0, 0]  Ts=1/fsw
      settings: LibrarySourceBlock=|
      | sps_lib/Sensors and Measurements/Power
      | (Positive-Sequence)
  Scope{,1..3} (4 alike) : Scope  NumInputPorts=2
  Scope{4,6..8} (4 alike) : Scope
  Scope5 : Scope  NumInputPorts=3
  Sum{,1..2,4,6} (5 alike) : Sum  Inputs=|+-
  Sum3 : Sum  Inputs=+|+|-
  Sum5 : Sum  Inputs=+|+
  Sum7 : Sum  Inputs=+|+|+
  dq0 to abc : spsdq0toabcLib/dq0 to abc  Alignment=90 degrees behind phase A axis
  gate : Outport
  wires:
  Constant/1 -> Mux/3
  PID Controller2/1 -> Sum5/2
  wt/1 -> dq0 to abc/2
  Mux/1 -> dq0 to abc/1
  Ud_ref/1 -> Scope/1, Sum/1
  Iq/1 -> Gain1/1, Sum6/2, Scope3/2
  Uq/1 -> Sum4/2, Scope1/2, Sum7/3, Gain3/1
  Sum3/1 -> Mux/1
  Sum5/1 -> Scope3/1, Sum6/1  "iq_ref"
  Sum2/1 -> PID Controller1/1
  Sum/1 -> PID Controller/1
  Sum7/1 -> Mux/2
  PID Controller1/1 -> Sum3/2  "Idef"
  Gain/1 -> Sum5/1
  Uq_ref/1 -> Scope1/1, Sum4/1
  Ud/1 -> Scope/2, Sum/2, Sum3/1, Gain/1
  Sum6/1 -> PID Controller3/1
  Sum4/1 -> PID Controller2/1
  Id/1 -> Gain4/1, Sum2/2, Scope2/2
  PID Controller3/1 -> Sum7/2  "Idef"
  PWM Generator (2-Level)/1 -> gate/1
  dq0 to abc/1 -> Gain2/1
  Gain2/1 -> Scope4/1, PWM Generator (2-Level)/1
  PID Controller/1 -> Sum1/1
  Gain3/1 -> Sum1/2
  Sum1/1 -> Scope2/1, Sum2/1
  Gain1/1 -> Sum3/3
  Gain4/1 -> Sum7/1
  PLL (3ph)/1 -> Scope8/1
  [Iabc] -> Power (Positive-Sequence)/2
  Demux3/1 -> Scope5/1
  Demux3/2 -> Scope5/2
  Power (Positive-Sequence)/1 -> Display1/1, Scope6/1
  [Uabc] -> PLL (3ph)/1, Power (Positive-Sequence)/1, Demux3/1
  Power (Positive-Sequence)/2 -> Display2/1, Scope7/1
  Demux3/3 -> Scope5/3

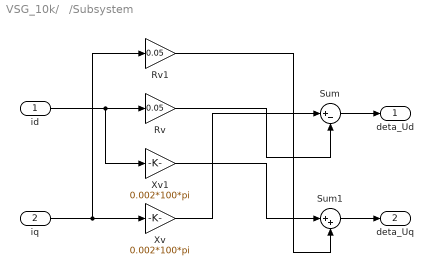
== system VSG_10k/   /Subsystem ==
  id : Inport
  iq : Inport  Port=2
  Rv : Gain  Gain=0.05
  Rv1 : Gain  Gain=0.05
  Sum : Sum  Inputs=|+-
  Sum1 : Sum  Inputs=|++
  Xv : Gain  Gain=0.002*100*pi
  Xv1 : Gain  Gain=0.002*100*pi
  deta_Ud : Outport
  deta_Uq : Outport  Port=2
  wires:
  Sum/1 -> deta_Ud/1
  Sum1/1 -> deta_Uq/1
  id/1 -> Xv1/1, Rv/1
  Rv/1 -> Sum/2
  iq/1 -> Rv1/1, Xv/1
  Xv/1 -> Sum/1
  Xv1/1 -> Sum1/1
  Rv1/1 -> Sum1/2
